simulink model "Unipolar_Hbridge_&_Filter"  (R2023a)
settings: Solver=VariableStepAuto  StartTime=0.0  StopTime=0.1  RelTol=1e-3
PreLoadFcn:
  | V_in = 350;
  | Fsw = 23400;
  | Vref = 230;
  | Fc = 50;
model workspace (MAT data in the model file):
  Vin = 400
  Vref = 230
libraries: spsSeriesRLCBranchLib x6, spsIGBTDiodeLib x4, spsVoltageMeasurementLib x2, spsDCVoltageSourceLib x1, simulink x1, sps_lib x1
settings Model: Creator=Rakesh  LastModifiedBy=Rakesh

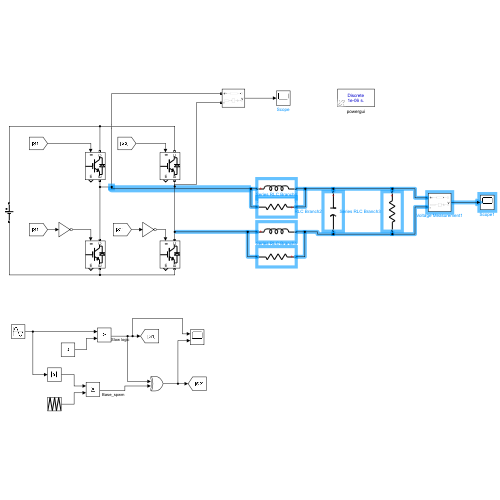
[thumbnail: Simulink's stored preview of the top-level diagram]
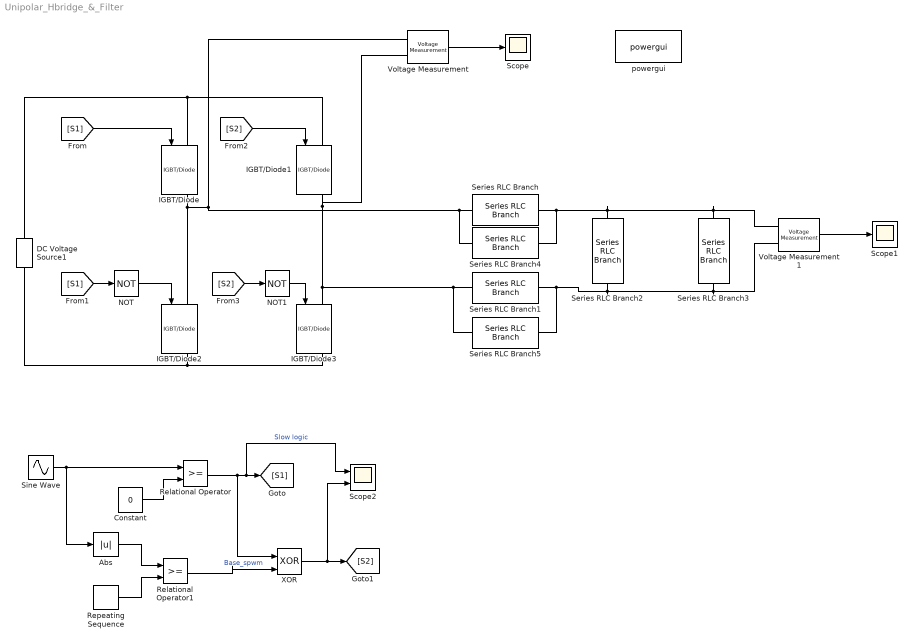
== system Unipolar_Hbridge_&_Filter ==
  Abs : Abs  SaturateOnIntegerOverflow=off
  Constant : Constant  Value=0  SampleTime=-1
  DC Voltage Source1 : spsDCVoltageSourceLib/DC Voltage Source  Amplitude=350  Measurements=None
  IGBT/Diode{,1..3} (4 alike) : spsIGBTDiodeLib/IGBT//Diode  Ron=1e-3  Rs=1e5  Cs=inf  Measurements=on
  NOT : Logic  Operator=NOT  IconShape=distinctive  AllPortsSameDT=off  OutDataTypeStr=boolean
  NOT1 : Logic  Operator=NOT  IconShape=distinctive  AllPortsSameDT=off  OutDataTypeStr=boolean
  Relational Operator : RelationalOperator  OutDataTypeStr=boolean  RndMeth=Simplest  InputSameDT=off
  Relational Operator1 : RelationalOperator  OutDataTypeStr=boolean  RndMeth=Simplest  InputSameDT=off
  Repeating Sequence : simulink/Sources/Repeating Sequence  rep_seq_t=[0 0.5/23400 1/23400]  rep_seq_y=[0 1.2 0]
  Scope : Scope
  Scope1 : Scope
  Scope2 : Scope  NumInputPorts=2
  Series RLC Branch : spsSeriesRLCBranchLib/Series RLC Branch  LConnTagsString=__new0  RConnTagsString=__new0  BranchType=L  Resistance=1  Inductance=890e-6  SetiL0=off  InitialCurrent=0  Capacitance=1e-6  Setx0=off  InitialVoltage=0  Measurements=None
  Series RLC Branch1 : spsSeriesRLCBranchLib/Series RLC Branch  LConnTagsString=__new0  RConnTagsString=__new0  BranchType=L  Resistance=1  Inductance=890e-6  SetiL0=off  InitialCurrent=0  Capacitance=1e-6  Setx0=off  InitialVoltage=0  Measurements=None
  Series RLC Branch2 : spsSeriesRLCBranchLib/Series RLC Branch  LConnTagsString=__new0  RConnTagsString=__new0  BranchType=C  Resistance=1  Inductance=890e-6  SetiL0=off  InitialCurrent=0  Capacitance=2e-6  Setx0=off  InitialVoltage=0  Measurements=None
  Series RLC Branch3 : spsSeriesRLCBranchLib/Series RLC Branch  LConnTagsString=__new0  RConnTagsString=__new0  BranchType=R  Resistance=180  Inductance=890e-6  SetiL0=off  InitialCurrent=0  Capacitance=1e-6  Setx0=off  InitialVoltage=0  Measurements=None
  Series RLC Branch4 : spsSeriesRLCBranchLib/Series RLC Branch  LConnTagsString=__new0  RConnTagsString=__new0  BranchType=R  Resistance=120  Inductance=890e-6  SetiL0=off  InitialCurrent=0  Capacitance=1e-6  Setx0=off  InitialVoltage=0  Measurements=None
  Series RLC Branch5 : spsSeriesRLCBranchLib/Series RLC Branch  LConnTagsString=__new0  RConnTagsString=__new0  BranchType=R  Resistance=120  Inductance=890e-6  SetiL0=off  InitialCurrent=0  Capacitance=1e-6  Setx0=off  InitialVoltage=0  Measurements=None
  Sine Wave : Sin  Frequency=2*pi*Fc  SampleTime=0
  Voltage Measurement : spsVoltageMeasurementLib/Voltage Measurement  PhasorSimulation=off  OutputType=Complex  PSBequivalent=0
  Voltage Measurement1 : spsVoltageMeasurementLib/Voltage Measurement  PhasorSimulation=off  OutputType=Complex  PSBequivalent=0
  XOR : Logic  Operator=XOR  IconShape=distinctive  AllPortsSameDT=off  OutDataTypeStr=boolean
  powergui : sps_lib/powergui  Priority=1  SimulationMode=Discrete  SampleTime=1e-6  frequency=60  Iterations=50  frequencyindice=0  Pbase=100e6  ErrMax=1e-4  UnitsV=kV  UnitsW=MW  buscounter=0  FunctionMessages=off  echomessages=off  EnableUseOfTLC=off  CurrentSourceSwitches=off  DisableSnubberDevices=off  DisableRonSwitches=off  DisableVfSwitches=off  DisplayEquations=off  AutomaticDiscreteSolvers=off  SolverType=Tustin/Backward Euler (TBE)  Interpol=off  ExternalGateDelay=off  methode=off  Ts=100  x0status=blocks  SPID=on  SwTol=0  HookPort=off  NonlinearTolerance=1e-4  nMaxIteration=100  ContinueOnMaxIteration=off  RestoreLinks=warning  ResistiveCurrentMeasurement=off  Frange=[0:2:500]  Ylog=off  Xlog=on  ShowGrid=off  save=off  variable=ZData  structure=0  ZoomFFT=off  StartTime=0.0  cycles=1  DisplayStyle=1  fundamental=60  FreqAxis=off  MaxFrequency=1000  frequencyindicesteady=1  RmsSteady=1  display=off
  wires:
  [S1] -> NOT/1
  [S2] -> NOT1/1
  [S1] -> IGBT/Diode/1
  NOT/1 -> IGBT/Diode2/1
  NOT1/1 -> IGBT/Diode3/1
  [S2] -> IGBT/Diode1/1
  Voltage Measurement/1 -> Scope/1
  Voltage Measurement1/1 -> Scope1/1
  Sine Wave/1 -> Abs/1, Relational Operator/1
  Constant/1 -> Relational Operator/2
  Abs/1 -> Relational Operator1/1
  Repeating Sequence/1 -> Relational Operator1/2
  Relational Operator/1 -> XOR/1, Scope2/1, [S1]  "Slow logic"
  Relational Operator1/1 -> XOR/2  "Base_spwm"
  XOR/1 -> Scope2/2, [S2]
  connections:
  IGBT/Diode1/LConn1 -- DC Voltage Source1/RConn1 -- IGBT/Diode/LConn1
  IGBT/Diode2/RConn1 -- DC Voltage Source1/LConn1 -- IGBT/Diode3/RConn1
  IGBT/Diode/RConn1 -- IGBT/Diode2/LConn1 -- Series RLC Branch4/RConn1 -- Series RLC Branch/LConn1 -- Voltage Measurement/LConn1
  IGBT/Diode1/RConn1 -- IGBT/Diode3/LConn1 -- Series RLC Branch5/RConn1 -- Series RLC Branch1/LConn1 -- Voltage Measurement/LConn2
  Series RLC Branch/RConn1 -- Series RLC Branch4/LConn1 -- Series RLC Branch3/LConn1 -- Voltage Measurement1/LConn1 -- Series RLC Branch2/LConn1
  Series RLC Branch1/RConn1 -- Series RLC Branch5/LConn1 -- Series RLC Branch2/RConn1 -- Series RLC Branch3/RConn1 -- Voltage Measurement1/LConn2
